simulink model "CruiseControl_TestGen_DisengageWithBrake_"  (R2018b)
settings: Solver=FixedStepDiscrete  StartTime=0.0  StopTime=2  FixedStep=0.1  RelTol=1e-3  EnableMultiTasking=on
undefined symbols (not defined in the file): sldvsubsys
libraries: sldvlib x3, simulink x1
settings Model: DataDictionary=CruiseControl_Req_dd.sldd  Creator=colosky  LastModifiedBy=colosky
settings DataIOCC: LimitDataPoints=on  SaveFormat=Array  SaveOutput=off  SaveTime=off
settings OptimizationCC: DefaultParameterBehavior=Inlined  InlineInvariantSignals=on  ExpressionDepthLimit=2147483647  InitFltsAndDblsToZero=on  NoFixptDivByZeroProtection=on  LifeSpan=inf
settings DebuggingCC: SignalInfNanChecking=warning  SaveWithParameterizedLinksMsg=none  UnderspecifiedInitializationDetection=Classic  MergeDetectMultiDrivingBlocksExec=none  SolverPrmCheckMsg=warning  FcnCallInpInsideContextMsg=warning  UniqueDataStoreMsg=warning  AllowSymbolicDim=off  StateNameClashWarn=warning  LibraryContextMissingDiagnostic=none  StrictBusMsg=ErrorOnBusTreatedAsVector  SFUnexpectedBacktrackingDiag=warning  SFNoUnconditionalDefaultTransitionDiag=warning  SFExecutionAtInitializationDiag=none
settings HardwareCC: ProdBitPerPointer=32  ProdBitPerSizeT=32  ProdBitPerPtrDiffT=32  ProdLargestAtomicFloat=None  ProdEndianess=Unspecified  ProdWordSize=32  ProdHWDeviceType=32-bit Generic
settings ModelReferenceCC: ModelReferenceNumInstancesAllowed=Single  PropagateSignalLabelsOutOfModel=off
settings SFSimCC: SimUseLocalCustomCode=off  SimParseCustomCode=off  MATLABDynamicMemAlloc=off
settings RTWCC: SystemTargetFile=ert.tlc  TemplateMakefile=ert_default_tmf  GenerateReport=on  RTWUseLocalCustomCode=off  IncludeHyperlinkInReport=on  LaunchReport=on  PortableWordSizes=on  GenerateTraceInfo=on  GenerateTraceReport=on  GenerateTraceReportSl=on  GenerateTraceReportSf=on  GenerateTraceReportEml=on
settings CodeAppCC: IgnoreCustomStorageClasses=off  CustomSymbolStrGlobalVar=$N$M  StateflowObjectComments=on
settings ERTTargetCC: MultiwordLength=2048  GenerateSampleERTMain=on  InlinedParameterPlacement=NonHierarchical  ERTCustomFileTemplate=example_file_process.tlc  ConvertIfToSwitch=off  SuppressUnreachableDefaultCases=off
settings ConfigComp: CovEnable=on  CovScope=ReferencedModels  RecordCoverage=on  CovMetricSettings=dcme  CovModelRefEnable=Off  CovExternalEMLEnable=off  CovSFcnEnable=off  DVMode=DesignErrorDetection  DVMaxProcessTime=3000  DVDisplayUnsatisfiableObjectives=on  DVAutomaticStubbing=off  DVMakeOutputFilesUnique=off  DVModelCoverageObjectives=None  DVMaxTestCaseSteps=500  DVTestSuiteOptimization=IndividualObjectives  DVAssertions=EnableAll  DVProofAssumptions=EnableAll  DVCoverageDataFile=CruiseControlCovManual.cvt  DVDetectDeadLogic=on  DVDetectActiveLogic=on  DVDetectIntegerOverflow=off  DVMaxViolationSteps=50  DVHarnessModelFileName=$ModelName$_harness_SLDV  DVReportIncludeGraphics=on  DVDisplayResultsOnModel=on  PSAutoStubLUT=off

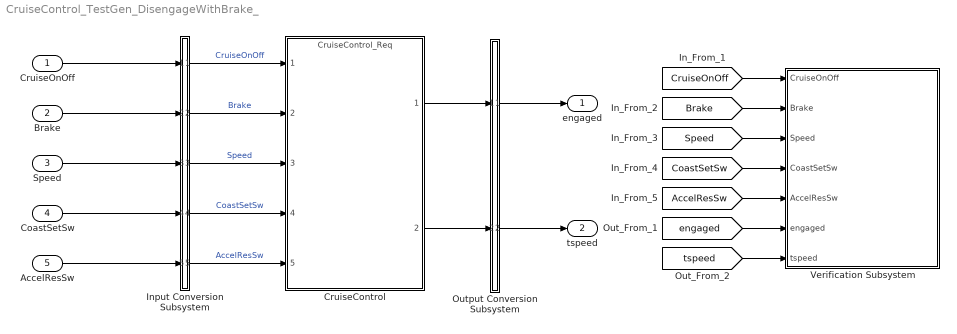
== system CruiseControl_TestGen_DisengageWithBrake_ ==
  CruiseOnOff : Inport  OutDataTypeStr=boolean  PortDimensions=[1]  SampleTime=0.1
  Brake : Inport  Port=2  OutDataTypeStr=boolean  PortDimensions=[1]  SampleTime=0.1
  Speed : Inport  Port=3  OutDataTypeStr=uint8  PortDimensions=[1]  SampleTime=0.1
  CoastSetSw : Inport  Port=4  OutDataTypeStr=boolean  PortDimensions=[1]  SampleTime=0.1
  AccelResSw : Inport  Port=5  OutDataTypeStr=boolean  PortDimensions=[1]  SampleTime=0.1
  CruiseControl : ModelReference  ModelNameDialog=CruiseControl_Req.slx  SimulationMode=Normal  ModelReferenceVersion=1.465
  Input Conversion Subsystem : Subsystem  Tag=__SLT_ICS__  Description=|
      | Signal spec.
      | and routing
      settings: AttributesFormatString=%<Description>
  Output Conversion Subsystem : Subsystem  Tag=__SLT_OCS__  Description=|
      | Signal spec.
      | and routing
      settings: AttributesFormatString=%<Description>
  Verification Subsystem : Subsystem  Tag=VerificationSubsystem  DisableCoverage=on  LoadFcn=sldvsubsys('check')  TreatAsAtomicUnit=on  SimViewingDevice=on  mask(VerificationSubsystem){}
      mask init:
      | sldvsubsys('maskInit');
      settings: CopyFcn=sldvsubsys('copy');  OpenFcn=open_system(gcb,'force');
      settings: PreSaveFcn=|
      | set_param(gcb,'SimViewingDevice','on');
      | sldvsubsys('check');
      mask Help: helpview(fullfile(docroot,'toolbox','sldv','sldv.map'),'verificationsubsystem')
      mask Display: image(imread('sldvicon_versubsys.png','BackGroundColor',[1 1 1]),'center');
  engaged : Outport  OutDataTypeStr=boolean  PortDimensions=[1]
  tspeed : Outport  Port=2  OutDataTypeStr=uint8  PortDimensions=[1]
  wires:
  CruiseOnOff/1 -> Input Conversion Subsystem/1(Inport_1)
  Brake/1 -> Input Conversion Subsystem/2(Inport_2)
  CoastSetSw/1 -> Input Conversion Subsystem/4(Inport_4)
  AccelResSw/1 -> Input Conversion Subsystem/5(Inport_5)
  Output Conversion Subsystem/1(Outport_1) -> engaged/1
  Output Conversion Subsystem/2(Outport_2) -> tspeed/1
  Input Conversion Subsystem/1(Outport_1) -> CruiseControl/1  "CruiseOnOff"
  Input Conversion Subsystem/2(Outport_2) -> CruiseControl/2  "Brake"
  Input Conversion Subsystem/3(Outport_3) -> CruiseControl/3  "Speed"
  Input Conversion Subsystem/4(Outport_4) -> CruiseControl/4  "CoastSetSw"
  Input Conversion Subsystem/5(Outport_5) -> CruiseControl/5  "AccelResSw"
  CruiseControl/1 -> Output Conversion Subsystem/1(Inport_1)
  CruiseControl/2 -> Output Conversion Subsystem/2(Inport_2)
  Speed/1 -> Input Conversion Subsystem/3(Inport_3)
  [CruiseOnOff] -> Verification Subsystem/1(CruiseOnOff)
  [Speed] -> Verification Subsystem/3(Speed)
  [AccelResSw] -> Verification Subsystem/5(AccelResSw)
  [engaged] -> Verification Subsystem/6(engaged)
  [Brake] -> Verification Subsystem/2(Brake)
  [tspeed] -> Verification Subsystem/7(tspeed)
  [CoastSetSw] -> Verification Subsystem/4(CoastSetSw)

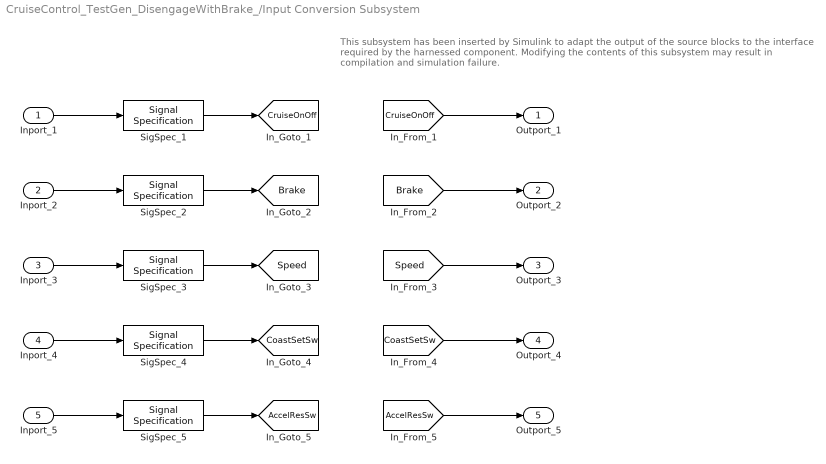
== system CruiseControl_TestGen_DisengageWithBrake_/Input Conversion Subsystem ==
  note: This subsystem has been inserted by Simulink to adapt the output of the source blocks to the interface required by the harnessed component.
      |  Modifying the contents of this subsystem may result in compilation and simulation failure.
  Inport_1 : Inport
  Inport_2 : Inport  Port=2
  Inport_3 : Inport  Port=3
  Inport_4 : Inport  Port=4
  Inport_5 : Inport  Port=5
  SigSpec_{1..2,4..5} (4 alike) : SignalSpecification  OutDataTypeStr=boolean  Dimensions=[1]  SampleTime=0.1
  SigSpec_3 : SignalSpecification  OutDataTypeStr=uint8  Dimensions=[1]  SampleTime=0.1
  Outport_1 : Outport
  Outport_2 : Outport  Port=2
  Outport_3 : Outport  Port=3
  Outport_4 : Outport  Port=4
  Outport_5 : Outport  Port=5
  tag scope: AccelResSw=global, Brake=global, CoastSetSw=global, CruiseOnOff=global, Speed=global
  wires:
  [CruiseOnOff] -> Outport_1/1
  SigSpec_1/1 -> [CruiseOnOff]
  Inport_1/1 -> SigSpec_1/1
  [Brake] -> Outport_2/1
  SigSpec_2/1 -> [Brake]
  Inport_2/1 -> SigSpec_2/1
  [Speed] -> Outport_3/1
  SigSpec_3/1 -> [Speed]
  Inport_3/1 -> SigSpec_3/1
  [CoastSetSw] -> Outport_4/1
  SigSpec_4/1 -> [CoastSetSw]
  Inport_4/1 -> SigSpec_4/1
  [AccelResSw] -> Outport_5/1
  SigSpec_5/1 -> [AccelResSw]
  Inport_5/1 -> SigSpec_5/1

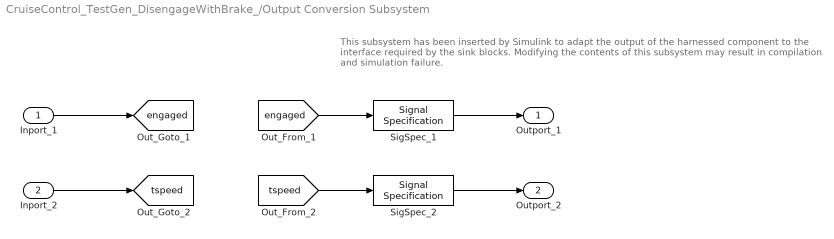
== system CruiseControl_TestGen_DisengageWithBrake_/Output Conversion Subsystem ==
  note: This subsystem has been inserted by Simulink to adapt the output of the harnessed component to the interface required by the sink blocks.
      |  Modifying the contents of this subsystem may result in compilation and simulation failure.
  Inport_1 : Inport
  Inport_2 : Inport  Port=2
  SigSpec_1 : SignalSpecification  OutDataTypeStr=boolean  Dimensions=[1]  SampleTime=0.1
  SigSpec_2 : SignalSpecification  OutDataTypeStr=uint8  Dimensions=[1]  SampleTime=0.1
  Outport_1 : Outport
  Outport_2 : Outport  Port=2
  tag scope: engaged=global, tspeed=global
  wires:
  Inport_1/1 -> [engaged]
  [engaged] -> SigSpec_1/1
  SigSpec_1/1 -> Outport_1/1
  Inport_2/1 -> [tspeed]
  [tspeed] -> SigSpec_2/1
  SigSpec_2/1 -> Outport_2/1

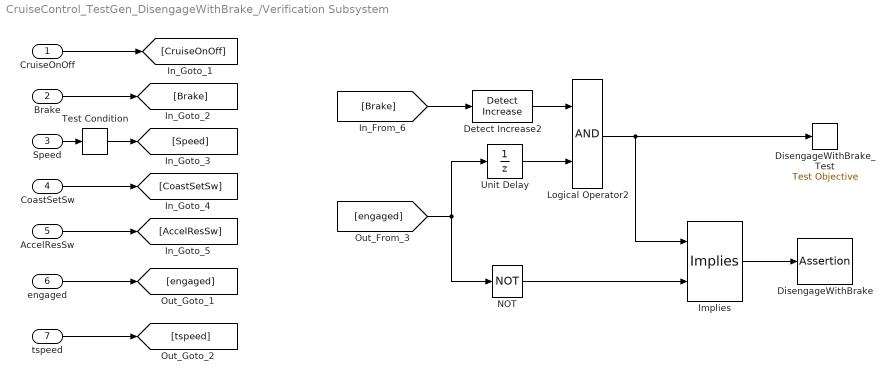
== system CruiseControl_TestGen_DisengageWithBrake_/Verification Subsystem ==
  CruiseOnOff : Inport  PortDimensions=1
  Brake : Inport  Port=2  PortDimensions=1
  Speed : Inport  Port=3  PortDimensions=1
  CoastSetSw : Inport  Port=4  PortDimensions=1
  AccelResSw : Inport  Port=5  PortDimensions=1
  engaged : Inport  Port=6  PortDimensions=1
  tspeed : Inport  Port=7  PortDimensions=1
  Detect Increase2 : simulink/Logic and Bit Operations/Detect Increase  vinit=false  OutDataTypeStr=boolean
  DisengageWithBrake : Assertion  StopWhenAssertionFail=off
  DisengageWithBrake_Test : sldvlib/Objectives and Constraints/Test Objective  enabled=on  customAVTBlockType=Test Objective  intervals=true  dispValues=on  outEnabled=off
      settings: AttributesFormatString=%<intervals>  SourceProductName=Simulink Design Verifier  SourceProductBaseCode=DV
  Implies : sldvlib/Verification Utilities/Implies
      settings: SourceProductName=Simulink Design Verifier  SourceProductBaseCode=DV
  Logical Operator2 : Logic  AllPortsSameDT=off  OutDataTypeStr=boolean
  NOT : Logic  Operator=NOT  AllPortsSameDT=off  OutDataTypeStr=boolean
  Test Condition : sldvlib/Objectives and Constraints/Test Condition  enabled=on  customAVTBlockType=Test Condition  intervals=[20, 90]  initial=off  dispValues=on  outEnabled=on
      settings: AttributesFormatString=%<intervals>  SourceProductName=Simulink Design Verifier  SourceProductBaseCode=DV
  Unit Delay : UnitDelay  SampleTime=-1
  wires:
  Unit Delay/1 -> Logical Operator2/2
  [Brake] -> Detect Increase2/1
  [engaged] -> NOT/1, Unit Delay/1
  Logical Operator2/1 -> Implies/1, DisengageWithBrake_Test/1
  Detect Increase2/1 -> Logical Operator2/1
  CoastSetSw/1 -> [CoastSetSw]
  Speed/1 -> Test Condition/1
  CruiseOnOff/1 -> [CruiseOnOff]
  Brake/1 -> [Brake]
  AccelResSw/1 -> [AccelResSw]
  engaged/1 -> [engaged]
  tspeed/1 -> [tspeed]
  Implies/1 -> DisengageWithBrake/1
  NOT/1 -> Implies/2
  Test Condition/1 -> [Speed]
